simulink model "simulator_acquisition_serial"  (Simulink 8.4)
settings: Solver=ode45  StartTime=0.0  StopTime=inf  RelTol=1e-3
libraries: aerolibfltsims x4
settings Model: Creator=AMANALLAH  LastModifiedBy=AMANALLAH
settings DataIOCC: SignalLoggingSaveFormat=Dataset
settings OptimizationCC: BlockReduction=off  ExpressionDepthLimit=128
settings DebuggingCC: UnderspecifiedInitializationDetection=Simplified  MergeDetectMultiDrivingBlocksExec=error  FcnCallInpInsideContextMsg=EnableAllAsError  StateNameClashWarn=none
settings GRTTargetCC: CombineOutputUpdateFcns=on  GRTInterface=off

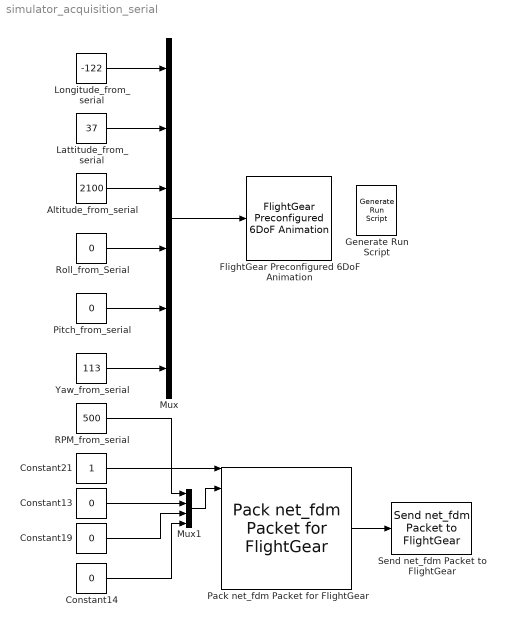
== system simulator_acquisition_serial ==
  Altitude_from_serial : Constant  Value=2100
  Constant13 : Constant  Value=0  OutDataTypeStr=single
  Constant14 : Constant  Value=0  OutDataTypeStr=single
  Constant19 : Constant  Value=0  OutDataTypeStr=single
  Constant21 : Constant  OutDataTypeStr=uint32
  FlightGear Preconfigured 6DoF Animation : aerolibfltsims/FlightGear Preconfigured 6DoF Animation  xFlightGearVersion=v3.0  DestinationIpAddress=127.0.0.1  DestinationPort=5502  SampleTime=1/30
  Generate Run Script : aerolibfltsims/Generate Run Script  OutputFileName=TA_test.bat  FlightGearBaseDirectory=C:\Program Files\FlightGear  GeometryModelName=spitfireIIa  DestinationPort=5502  OriginAddress=127.0.0.1  OriginPort=5505  LocalAddress=127.0.0.1  AirportId=KSFO  RunwayId=10L  InitialAltitude=7224  InitialHeading=113  OffsetDistance=4.72  OffsetAzimuth=0  GenerateFile=off  Architecture=Default  dataFlow=Send
  Lattitude_from_serial : Constant  Value=37
  Longitude_from_serial : Constant  Value=-122
  Mux : Mux  Inputs=6
  Mux1 : Mux
  Pack net_fdm Packet for FlightGear : aerolibfltsims/Pack net_fdm Packet for FlightGear  FlightGearVersion=v3.0  ShowPositionAttitudeInputs=off  ShowVelocityAccelerationInputs=off  ShowControlSurfacePositionInputs=off  ShowEngineFuelInputs=on  ShowLandingGearInputs=off  ShowEnvironmentInputs=off  SampleTime=1/30
  Pitch_from_serial : Constant  Value=0  OutDataTypeStr=double
  RPM_from_serial : Constant  Value=500  OutDataTypeStr=single
  Roll_from_Serial : Constant  Value=0  OutDataTypeStr=double
  Send net_fdm Packet to FlightGear : aerolibfltsims/Send net_fdm Packet to FlightGear  DestinationIpAddress=127.0.0.1  DestinationPort=5502  LocalIpPort=-1  varLen=off  SampleTime=1/30
  Yaw_from_serial : Constant  Value=113  OutDataTypeStr=double
  wires:
  Pack net_fdm Packet for FlightGear/1 -> Send net_fdm Packet to FlightGear/1
  RPM_from_serial/1 -> Mux1/1
  Constant13/1 -> Mux1/2
  Constant19/1 -> Mux1/3
  Constant14/1 -> Mux1/4
  Constant21/1 -> Pack net_fdm Packet for FlightGear/1
  Mux1/1 -> Pack net_fdm Packet for FlightGear/3
  Mux/1 -> FlightGear Preconfigured 6DoF Animation/1
  Longitude_from_serial/1 -> Mux/1
  Lattitude_from_serial/1 -> Mux/2
  Altitude_from_serial/1 -> Mux/3
  Roll_from_Serial/1 -> Mux/4
  Pitch_from_serial/1 -> Mux/5
  Yaw_from_serial/1 -> Mux/6
